simulink model "model_FS_PSH_IEEE39"  (R2020b)
settings: Solver=ode3  StartTime=0.0  StopTime=300  FixedStep=Ts  RelTol=1e-3
PostLoadFcn:
  | IEEE39BusLineLength;
  | vNomHV = 345E3;fNom=60;load('Dynamicload.mat');
InitFcn:
  | IEEE39BusLineLength;
  | vNomHV = 345E3;fNom=60;load('Dynamicload.mat');
values from neighbouring files (symbols this model uses):
  Rp = 0.05    [IEEE39BusLineLength.m]
  t_sw_off = 220    [MAIN_FS_PSH_IEEE39.m]    (also in MAIN_T_PSH_IEEE39.m; MAIN_VS_PSH.m = 45)
  t_sw_on = 130    [MAIN_FS_PSH_IEEE39.m]    (also in MAIN_T_PSH_IEEE39.m; MAIN_VS_PSH.m = 35)
  TL_10_11_len = 14    [IEEE39BusLineLength.m]
  TL_10_13_len = 14    [IEEE39BusLineLength.m]
  TL_13_14_len = 32    [IEEE39BusLineLength.m]
  TL_14_15_len = 70    [IEEE39BusLineLength.m]
  TL_15_16_len = 31.5    [IEEE39BusLineLength.m]
  TL_16_17_len = 26    [IEEE39BusLineLength.m]
  TL_16_19_len = 61    [IEEE39BusLineLength.m]
  TL_16_21_len = 46    [IEEE39BusLineLength.m]
  TL_16_24_len = 15    [IEEE39BusLineLength.m]
  TL_17_18_len = 26    [IEEE39BusLineLength.m]
  TL_17_27_len = 59    [IEEE39BusLineLength.m]
  TL_1_2_len = 134    [IEEE39BusLineLength.m]
  TL_1_39_len = 105    [IEEE39BusLineLength.m]
  TL_21_22_len = 47    [IEEE39BusLineLength.m]
  TL_22_23_len = 33    [IEEE39BusLineLength.m]
  TL_24_23_len = 88    [IEEE39BusLineLength.m]
  TL_25_26_len = 101    [IEEE39BusLineLength.m]
  TL_26_27_len = 46.5    [IEEE39BusLineLength.m]
  TL_26_28_len = 151    [IEEE39BusLineLength.m]
  TL_26_29_len = 200    [IEEE39BusLineLength.m]
  TL_28_29_len = 48    [IEEE39BusLineLength.m]
  TL_2_25_len = 28    [IEEE39BusLineLength.m]
  TL_2_2_len = 49    [IEEE39BusLineLength.m]
  TL_3_18_len = 42    [IEEE39BusLineLength.m]
  TL_3_4_len = 53    [IEEE39BusLineLength.m]
  TL_4_14_len = 33    [IEEE39BusLineLength.m]
  TL_4_5_len = 32.5    [IEEE39BusLineLength.m]
  TL_5_6_len = 14    [IEEE39BusLineLength.m]
  TL_5_8_len = 32    [IEEE39BusLineLength.m]
  TL_6_11_len = 26.5    [IEEE39BusLineLength.m]
  TL_6_7_len = 25.5    [IEEE39BusLineLength.m]
  TL_7_8_len = 15    [IEEE39BusLineLength.m]
  TL_8_9_len = 93    [IEEE39BusLineLength.m]
  TL_9_39_len = 136    [IEEE39BusLineLength.m]
  Ts = 25e-6    (= 2.5e-05)    [MAIN_FS_PSH_IEEE39.m]    (also in MAIN_T_PSH_IEEE39.m; MAIN_VS_PSH.m = 1e-07)
undefined symbols (not defined in the file or in its folder): D1, Delta, FS_PSH, load15, load16, load18, load20, load21, load23, load24, load25, load26, load27, load28, load29, load3, load39, load4, load7, load8
libraries: powerlib x216, sps_avr x10, powerlib_meascontrol x5, pid_lib x1
(part 3 of 8)

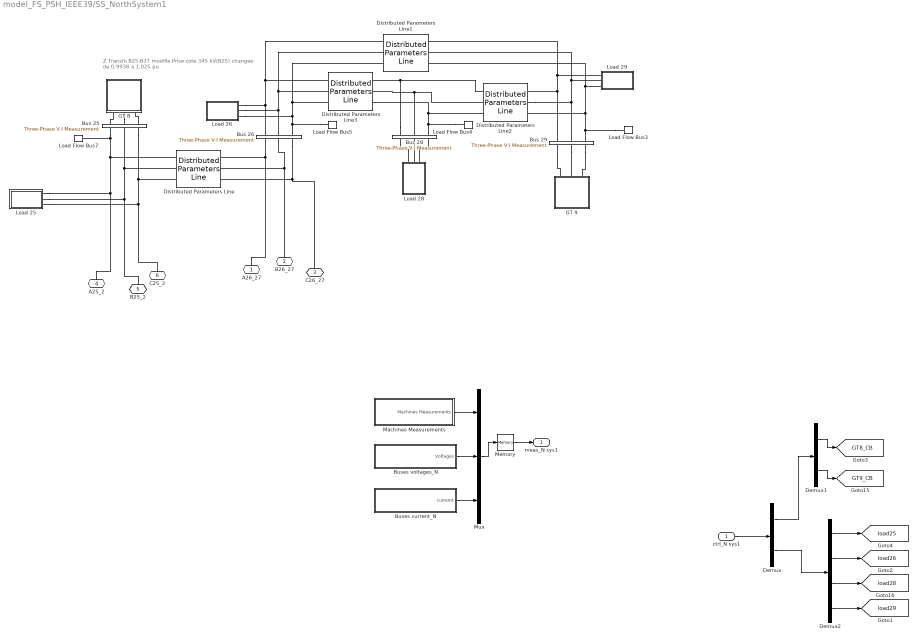
== system model_FS_PSH_IEEE39/SS_NorthSystem1 ==
  note: Z Transfo B25-B37 modifie
      | Prise cote 345 kV(B25)  changee de 0.9938 a 1.025 pu
  ctrl_N sys1 : Inport
  Bus 25 : powerlib/Measurements/Three-Phase V-I Measurement  VoltageMeasurement=phase-to-ground  SetLabelV=on  LabelV=V_bus_25  Vpu=off  VpuLL=off  CurrentMeasurement=yes  SetLabelI=on  LabelI=I_bus_25  Ipu=off  Pbase=100e6  Vbase=230e3  OutputType=Complex  PhasorSimulation=off  PSBequivalent=0
  Bus 26 : powerlib/Measurements/Three-Phase V-I Measurement  VoltageMeasurement=phase-to-ground  SetLabelV=on  LabelV=V_bus_26  Vpu=off  VpuLL=off  CurrentMeasurement=yes  SetLabelI=on  LabelI=I_bus_26  Ipu=off  Pbase=100e6  Vbase=230e3  OutputType=Complex  PhasorSimulation=off  PSBequivalent=0
  Bus 28 : powerlib/Measurements/Three-Phase V-I Measurement  VoltageMeasurement=phase-to-ground  SetLabelV=on  LabelV=V_bus_28  Vpu=off  VpuLL=off  CurrentMeasurement=yes  SetLabelI=on  LabelI=I_bus_28  Ipu=off  Pbase=100e6  Vbase=230e3  OutputType=Complex  PhasorSimulation=off  PSBequivalent=0
  Bus 29 : powerlib/Measurements/Three-Phase V-I Measurement  VoltageMeasurement=phase-to-ground  SetLabelV=on  LabelV=V_bus_29  Vpu=off  VpuLL=off  CurrentMeasurement=yes  SetLabelI=on  LabelI=I_bus_29  Ipu=off  Pbase=100e6  Vbase=230e3  OutputType=Complex  PhasorSimulation=off  PSBequivalent=0
  Buses current_N : Subsystem
  Buses voltages_N : Subsystem
  Demux : Demux  Outputs=[2 8]
  Demux1 : Demux  Outputs=2
  Demux2 : Demux  Outputs=[2 2 2 2]
  Distributed Parameters Line : powerlib/Elements/Distributed Parameters Line  Phases=3  Length=TL_25_26_len  Frequency=fNom  Resistance=[3.809 15.235]/TL_25_26_len  Inductance=[0.102 0.306]/TL_25_26_len  Capacitance=[1.143e-6 0.52e-6]/TL_25_26_len  x1=[-0.0004 -6.49801584942767e-10 0 0;-0.000375 -8.85176084526775e-10 0 0;-0.00035 -1.12047195765278e-09 197383.270025003 -196757.128056257;-0.000325 -1.35566830398082e-09 199228.856843478 -194888.123638832;-0.0003 -1.59074423201149e-09 201056.747002927 -193001.808131403;-0.000275 -1.82567886094164e-09 202866.778139577 -191098.349087419;-0.00025 -2.06045132251909e-09 204658.789475997 -189177.91558312;-0.000225 -2.29504076289635e-09 206432.621835377 -187240.678202513;-0.0002 -2.52942634448289e-09 208188.117655672 -185286.809022224;-0.000175 -2.76358724779611e-09 209925.121003593 -183316.481596211;-0.00015 -2.99750267331064e-09 211643.477588457 -181329.870940347;-0.000125 -3.23115184330587e-09 213343.034775899 -179327.15351688;-0.0001 -3.46451400371154e-09 215023.64160142 -177308.507218749;-7.5e-05 -3.69756842595122e-09 216685.148783807 -175274.111353792;-5e-05 -3.9302944087836e-09 218327.408738383 -173224.146628811;-2.5e-05 -4.16267128014124e-09 219950.275590124 -171158.795133528]  x2=[-0.0004 1.03117190872813e-08 0 0;-0.000375 1.00094674364182e-08 0 0;-0.00035 9.70632668678163e-09 176190.92375866 -212314.939973436;-0.000325 9.40232376508578e-09 178184.078450182 -210644.974463217;-0.0003 9.09748567462794e-09 180161.405801578 -208956.298248395;-0.000275 8.79183949288991e-09 182122.7301752 -207249.061326957;-0.00025 8.48541236913282e-09 184067.877354875 -205523.415345556;-0.000225 8.17823152198559e-09 185996.674561385 -203779.513586048;-0.0002 7.87032423702723e-09 187908.950467809 -202017.510951869;-0.000175 7.56171786436313e-09 189804.535214744 -200237.563954282;-0.00015 7.2524398161957e-09 191683.260425392 -198439.830698471;-0.000125 6.94251756438947e-09 193544.959220518 -196624.470869499;-0.0001 6.63197863803083e-09 195389.466233269 -194791.645718121;-7.5e-05 6.3208506209828e-09 197216.617623868 -192941.518046466;-5e-05 6.00916114943481e-09 199026.251094163 -191074.25219357;-2.5e-05 5.69693790944797e-09 200818.205902046 -189190.014020785]  x3=[-0.0004 7.28520624206915e-11 0 0;-0.000375 7.33520617392959e-11 0 0;-0.00035 7.38455455036475e-11 159.359042835864 -190.278599490576;-0.000325 7.43324698796652e-11 161.14522515065 -188.768251634971;-0.0003 7.48127916159104e-11 162.917093614779 -187.241136291779;-0.000275 7.52864680474291e-11 164.674490840651 -185.697389108214;-0.00025 7.5753457099542e-11 166.417260726082 -184.137147208828;-0.000225 7.62137172915813e-11 168.145248468174 -182.560549183328;-0.0002 7.66672077405753e-11 169.858300577064 -180.967735074265;-0.000175 7.71138881648803e-11 171.55626488956 -179.3588463646;-0.00015 7.75537188877582e-11 173.238990582652 -177.734025965129;-0.000125 7.79866608409012e-11 174.906328186915 -176.093418201797;-0.0001 7.84126755679015e-11 176.558129599783 -174.43716880287;-7.5e-05 7.8831725227668e-11 178.194248098704 -172.765424885996;-5e-05 7.92437725977868e-11 179.81453835417 -171.078334945138;-2.5e-05 7.9648781077828e-11 181.418856442635 -169.376048837377]  x4=[-0.0004 -5.6133067329239e-11 0 0;-0.000375 -5.73097615568789e-11 0 0;-0.00035 -5.84813652001265e-11 991.580164096685 -1246.13955007551;-0.000325 -5.9647774190372e-11 1003.28050960891 -1236.73892106488;-0.0003 -6.08088849204244e-11 1014.8917379452 -1227.22843775233;-0.000275 -6.19645942537151e-11 1026.41281772913 -1217.60894491398;-0.00025 -6.31147995334587e-11 1037.84272559176 -1207.88129700881;-0.000225 -6.42593985917716e-11 1049.18044626259 -1198.04635810275;-0.0002 -6.53982897587474e-11 1060.42497265972 -1188.10500179193;-0.000175 -6.65313718714872e-11 1071.57530597929 -1178.05811112512;-0.00015 -6.76585442830864e-11 1082.63045578423 -1167.90657852522;-0.000125 -6.87797068715739e-11 1093.58944009221 -1157.65130571007;-0.0001 -6.98947600488058e-11 1104.45128546288 -1147.29320361229;-7.5e-05 -7.10036047693117e-11 1115.21502708433 -1136.83319229839;-5e-05 -7.2106142539092e-11 1125.87970885878 -1126.27220088708;-2.5e-05 -7.3202275424367e-11 1136.44438348754 -1115.61116746666]  x5=0.000398898483326272  V1=ones(3,3)  V2=ones(3,3)  I1=ones(3,3)  I2=ones(3,3)  nHarmo=1  Measurements=None  Decoupling=off  VsMag0=0  VrMag0=0  VsAngle0=0  VrAngle0=0  IsMag0=0  IrMag0=0  IsAngle0=0  IrAngle0=0
  Distributed Parameters Line1 : powerlib/Elements/Distributed Parameters Line  Phases=3  Length=TL_26_29_len  Frequency=fNom  Resistance=[6.784 27.138]/TL_26_29_len  Inductance=[0.197 0.592]/TL_26_29_len  Capacitance=[2.293e-6 1.043e-6]/TL_26_29_len  x1=[-0.0008 1.50051894992801e-08 0 0;-0.000775 1.47207537868238e-08 0 0;-0.00075 1.44350104918993e-08 0 0;-0.000725 1.41479849958782e-08 0 0;-0.0007 1.38597027940247e-08 0 0;-0.000675 1.35701894932309e-08 148922.028977619 -232256.649579684;-0.00065 1.3279470809742e-08 151104.338220983 -230842.799306395;-0.000625 1.29875725668726e-08 153273.225503325 -229408.444240916;-0.0006 1.26945206927124e-08 155428.498171536 -227953.711790957;-0.000575 1.24003412178233e-08 157569.964781837 -226478.731174265;-0.00055 1.21050602729271e-08 159697.435116781 -224983.633407148;-0.000525 1.18087040865849e-08 161810.720202151 -223468.551292834;-0.0005 1.15112989828666e-08 163909.632323747 -221933.619409676;-0.000475 1.12128713790131e-08 165993.985044058 -220378.974099199;-0.00045 1.09134477830898e-08 168063.593218823 -218804.75345399;-0.000425 1.06130547916317e-08 170118.273013478 -217211.097305428;-0.0004 1.03117190872813e-08 172157.841919484 -215598.147211267;-0.000375 1.00094674364182e-08 174182.118770535 -213966.046443061;-0.00035 9.70632668678163e-09 176190.92375866 -212314.939973436;-0.000325 9.40232376508578e-09 178184.078450182 -210644.974463217;-0.0003 9.09748567462794e-09 180161.405801578 -208956.298248395;-0.000275 8.79183949288991e-09 182122.7301752 -207249.061326957;-0.00025 8.48541236913282e-09 184067.877354875 -205523.415345556;-0.000225 8.17823152198559e-09 185996.674561385 -203779.513586048;-0.0002 7.87032423702723e-09 187908.950467809 -202017.510951869;-0.000175 7.56171786436313e-09 189804.535214744 -200237.563954282;-0.00015 7.2524398161957e-09 191683.260425392 -198439.830698471;-0.000125 6.94251756438947e-09 193544.959220518 -196624.470869499;-0.0001 6.63197863803083e-09 195389.466233269 -194791.645718121;-7.5e-05 6.3208506209828e-09 197216.617623868 -192941.518046466;-5e-05 6.00916114943481e-09 199026.251094163 -191074.25219357;-2.5e-05 5.69693790944797e-09 200818.205902046 -189190.014020785]  x2=[-0.0008 7.55362211098819e-09 0 0;-0.000775 7.10605204161126e-09 0 0;-0.00075 6.65785077160409e-09 0 0;-0.000725 6.20905811279503e-09 0 0;-0.0007 5.75971392954299e-09 0 0;-0.000675 5.30985813519648e-09 172202.954349061 -215442.997241187;-0.00065 4.85953068854828e-09 174225.766489807 -213810.479094855;-0.000625 4.40877159028602e-09 176233.102890582 -212158.969065496;-0.0006 3.95762087943915e-09 178224.785248162 -210488.613849781;-0.000575 3.50611862982241e-09 180200.636649801 -208799.561818317;-0.00055 3.05430494647624e-09 182160.481588956 -207091.963002472;-0.000525 2.60221996210443e-09 184104.145980865 -205365.969081047;-0.0005 2.14990383350928e-09 186031.45717802 -203621.733366801;-0.000475 1.69739673802468e-09 187942.243985496 -201859.410792836;-0.00045 1.2447388699473e-09 189836.33667616 -200079.157898834;-0.000425 7.91970436966276e-10 191713.567005747 -198281.132817149;-0.0004 3.39131656591792e-10 193573.768227806 -196465.495258766;-0.000375 -1.13737247417326e-10 195416.775108509 -194632.40649911;-0.00035 -5.66596048626487e-10 197242.423941326 -192782.029363726;-0.000325 -1.01940452149849e-09 199050.552561574 -190914.528213808;-0.0003 -1.4721224449666e-09 200841.000360813 -189030.068931607;-0.000275 -1.92470960600719e-09 202613.608301116 -187128.818905693;-0.00025 -2.3771258032117e-09 204368.218929199 -185210.947016086;-0.000225 -2.8293308503576e-09 206104.676390398 -183276.623619257;-0.0002 -3.28128457997789e-09 207822.826442523 -181326.020532994;-0.000175 -3.73294684692907e-09 209522.516469551 -179359.311021142;-0.00015 -4.18427753195704e-09 211203.595495185 -177376.669778212;-0.000125 -4.6352365452607e-09 212865.914196267 -175378.272913863;-0.0001 -5.08578383005301e-09 214509.324916039 -173364.297937258;-7.5e-05 -5.53587936611902e-09 216133.681677256 -171334.923741301;-5e-05 -5.98548317337072e-09 217738.840195161 -169290.330586741;-2.5e-05 -6.4345553153983e-09 219324.657890292 -167230.700086165]  x3=[-0.0008 9.67658806424509e-11 0 0;-0.000775 9.60264170672028e-11 0 0;-0.00075 9.52784238703564e-11 0 0;-0.000725 9.45219674929924e-11 0 0;-0.0007 9.37571151279402e-11 0 0;-0.000675 9.29839347138093e-11 651.879190253851 -1133.09716308397;-0.00065 9.22024949289546e-11 662.529226151143 -1126.90312906639;-0.000625 9.14128651853763e-11 673.120412371758 -1120.60899699703;-0.0006 9.06151156225538e-11 683.651808145296 -1114.21532595707;-0.000575 8.98093171012161e-11 694.122478012292 -1107.72268386936;-0.00055 8.89955411970469e-11 704.531491907304 -1101.1316474479;-0.000525 8.81738601943275e-11 714.877925241533 -1094.44280214666;-0.0005 8.73443470795155e-11 725.160858984947 -1087.65674210756;-0.000475 8.6507075534762e-11 735.379379747913 -1080.77407010768;-0.00045 8.56621199313671e-11 745.532579862332 -1073.79539750575;-0.000425 8.48095553231728e-11 755.619557462263 -1066.72134418783;-0.0004 8.39494574398973e-11 765.639416564033 -1059.55253851222;-0.000375 8.30819026804079e-11 775.591267145819 -1052.2896172537;-0.00035 8.22069681059345e-11 785.474225226711 -1044.93322554693;-0.000325 8.1324731433225e-11 795.287412945228 -1037.48401682917;-0.0003 8.04352710276418e-11 805.029958637294 -1029.94265278218;-0.000275 7.95386658962011e-11 814.700996913671 -1022.30980327355;-0.00025 7.8634995680555e-11 824.299668736819 -1014.5861462971;-0.000225 7.77243406499171e-11 833.825121497207 -1006.77236791269;-0.0002 7.68067816939327e-11 843.276509089042 -998.869162185301;-0.000175 7.58824003154938e-11 852.652991985431 -990.877231123367;-0.00015 7.49512786234991e-11 861.953737312946 -982.797284616414;-0.000125 7.40134993255613e-11 871.17791892561 -974.630040372008;-0.0001 7.306914572066e-11 880.324717478277 -966.376223852008;-7.5e-05 7.21183016917425e-11 889.393320499412 -958.036568208121;-5e-05 7.11610516982736e-11 898.382922463258 -949.611814216781;-2.5e-05 7.01974807687325e-11 907.292724861391 -941.102710213353]  x4=[-0.0008 -5.32627553331173e-11 0 0;-0.000775 -5.34322521881827e-11 0 0;-0.00075 -5.3597002881658e-11 0 0;-0.000725 -5.37569927794341e-11 0 0;-0.0007 -5.39122076702832e-11 0 0;-0.000675 -5.40626337671213e-11 232.453391057633 -505.849442519053;-0.00065 -5.42082577082325e-11 237.210479576283 -503.636188539323;-0.000625 -5.43490665584566e-11 241.946497688563 -501.378198681252;-0.0006 -5.44850478103371e-11 246.66102471396 -499.075673512555;-0.000575 -5.46161893852332e-11 251.353641880922 -496.728817556831;-0.00055 -5.47424796343917e-11 256.023932364061 -494.337839275396;-0.000525 -5.48639073399826e-11 260.671481321171 -491.902951048765;-0.0005 -5.4980461716095e-11 265.295875930081 -489.42436915779;-0.000475 -5.50921324096952e-11 269.896705425324 -486.902313764445;-0.00045 -5.51989095015465e-11 274.473561134621 -484.337008892274;-0.000425 -5.53007835070902e-11 279.026036515185 -481.728682406488;-0.0004 -5.53977453772882e-11 283.553727189828 -479.077565993727;-0.000375 -5.54897864994264e-11 288.056230982887 -476.383895141479;-0.00035 -5.55768986978802e-11 292.533147955939 -473.647909117166;-0.000325 -5.56590742348405e-11 296.984080443334 -470.869850946885;-0.0003 -5.57363058110009e-11 301.408633087513 -468.049967393826;-0.000275 -5.58085865662062e-11 305.806412874125 -465.188508936352;-0.00025 -5.58759100800619e-11 310.177029166943 -462.285729745747;-0.000225 -5.59382703725042e-11 314.520093742555 -459.341887663643;-0.0002 -5.59956619043312e-11 318.835220824855 -456.357244179117;-0.000175 -5.60480795776954e-11 323.122027119303 -453.332064405459;-0.00015 -5.60955187365559e-11 327.380131846979 -450.266617056629;-0.000125 -5.61379751670922e-11 331.609156778399 -447.161174423385;-0.0001 -5.61754450980789e-11 335.808726267117 -444.016012349098;-7.5e-05 -5.62079252012198e-11 339.978467283088 -440.831410205249;-5e-05 -5.62354125914445e-11 344.118009445805 -437.607650866615;-2.5e-05 -5.62579048271641e-11 348.226985057198 -434.345020686138]  x5=0.000785783685246773  V1=ones(3,3)  V2=ones(3,3)  I1=ones(3,3)  I2=ones(3,3)  nHarmo=1  Measurements=None  Decoupling=off  VsMag0=0  VrMag0=0  VsAngle0=0  VrAngle0=0  IsMag0=0  IrMag0=0  IsAngle0=0  IrAngle0=0
  Distributed Parameters Line2 : powerlib/Elements/Distributed Parameters Line  Phases=3  Length=TL_28_29_len  Frequency=fNom  Resistance=[1.666 6.665]/TL_28_29_len  Inductance=[0.048 0.143]/TL_28_29_len  Capacitance=[0.555e-6 0.252e-6]/TL_28_29_len  x1=[-0.0002 -1.22627753912243e-09 0 0;-0.000175 -1.67405795565669e-09 199382.259554779 -190507.622683492;-0.00015 -2.12168967268375e-09 201168.857786666 -188620.054664454;-0.000125 -2.56913292896627e-09 202937.587037427 -186715.732321541;-0.0001 -3.01634798000704e-09 204688.290198301 -184794.824807674;-7.5e-05 -3.46329510157941e-09 206420.811761712 -182857.502748965;-5e-05 -3.90993459325574e-09 208134.997835076 -180903.938229561;-2.5e-05 -4.35622678193386e-09 209830.696154475 -178934.30477636]  x2=[-0.0002 -3.28128457997789e-09 0 0;-0.000175 -3.73294684692907e-09 209522.516469551 -179359.311021142;-0.00015 -4.18427753195704e-09 211203.595495185 -177376.669778212;-0.000125 -4.6352365452607e-09 212865.914196267 -175378.272913863;-0.0001 -5.08578383005301e-09 214509.324916039 -173364.297937258;-7.5e-05 -5.53587936611902e-09 216133.681677256 -171334.923741301;-5e-05 -5.98548317337072e-09 217738.840195161 -169290.330586741;-2.5e-05 -6.4345553153983e-09 219324.657890292 -167230.700086165]  x3=[-0.0002 2.67643326896294e-12 0 0;-0.000175 1.71222017251387e-12 1315.78655166209 -1164.2244305845;-0.00015 7.47854986768843e-13 1326.70046147759 -1151.77191008628;-0.000125 -2.16576627780281e-13 1337.49652608699 -1139.21708254734;-0.0001 -1.18098900474106e-12 1348.1737865214 -1126.56106316006;-7.5e-05 -2.14529647942984e-12 1358.73129436482 -1113.80497610527;-5e-05 -3.10941339648099e-12 1369.16811183835 -1100.94995445236;-2.5e-05 -4.07325411745533e-12 1379.48331188352 -1087.9971400587]  x4=[-0.0002 -5.82099425675479e-12 0 0;-0.000175 -6.07694386964931e-12 30.1483729405909 -130.796513455747;-0.00015 -6.33235369325182e-12 31.3797081394057 -130.506561579167;-0.000125 -6.587201040585e-12 32.608256011103 -130.205017355186;-0.0001 -6.84146327463389e-12 33.8339074289571 -129.891907568706;-7.5e-05 -7.0951178103567e-12 35.0565535235224 -129.567260031946;-5e-05 -7.34814211669091e-12 36.2760856923032 -129.23110358198;-2.5e-05 -7.60051371855463e-12 37.4923956094008 -128.883468078167]  x5=0.000189831504234676  V1=ones(3,3)  V2=ones(3,3)  I1=ones(3,3)  I2=ones(3,3)  nHarmo=1  Measurements=None  Decoupling=off  VsMag0=0  VrMag0=0  VsAngle0=0  VrAngle0=0  IsMag0=0  IrMag0=0  IsAngle0=0  IrAngle0=0
  Distributed Parameters Line3 : powerlib/Elements/Distributed Parameters Line  Phases=3  Length=TL_26_28_len  Frequency=fNom  Resistance=[5.118 20.472]/TL_26_28_len  Inductance=[0.15 0.449]/TL_26_28_len  Capacitance=[1.739e-6 0.791e-6]/TL_26_28_len  x1=[-0.0006 1.26945206927124e-08 0 0;-0.000575 1.24003412178233e-08 0 0;-0.00055 1.21050602729271e-08 0 0;-0.000525 1.18087040865849e-08 161810.720202151 -223468.551292834;-0.0005 1.15112989828666e-08 163909.632323747 -221933.619409676;-0.000475 1.12128713790131e-08 165993.985044058 -220378.9740992;-0.00045 1.09134477830898e-08 168063.593218823 -218804.75345399;-0.000425 1.06130547916317e-08 170118.273013478 -217211.097305428;-0.0004 1.03117190872813e-08 172157.841919484 -215598.147211267;-0.000375 1.00094674364182e-08 174182.118770535 -213966.046443061;-0.00035 9.70632668678163e-09 176190.92375866 -212314.939973436;-0.000325 9.40232376508578e-09 178184.078450182 -210644.974463217;-0.0003 9.09748567462794e-09 180161.405801578 -208956.298248395;-0.000275 8.79183949288991e-09 182122.7301752 -207249.061326957;-0.00025 8.48541236913282e-09 184067.877354875 -205523.415345556;-0.000225 8.17823152198559e-09 185996.674561385 -203779.513586048;-0.0002 7.87032423702723e-09 187908.950467809 -202017.510951869;-0.000175 7.56171786436313e-09 189804.535214744 -200237.563954282;-0.00015 7.2524398161957e-09 191683.260425392 -198439.830698471;-0.000125 6.94251756438947e-09 193544.959220518 -196624.470869499;-0.0001 6.63197863803083e-09 195389.466233269 -194791.645718121;-7.5e-05 6.3208506209828e-09 197216.617623868 -192941.518046466;-5e-05 6.00916114943481e-09 199026.251094163 -191074.25219357;-2.5e-05 5.69693790944797e-09 200818.205902046 -189190.014020785]  x2=[-0.0006 5.92679287461096e-09 0 0;-0.000575 5.48200731026818e-09 0 0;-0.00055 5.03673480233859e-09 0 0;-0.000525 4.59101490250095e-09 172585.310861128 -215083.277740955;-0.0005 4.14488720217396e-09 174604.715817765 -213447.171400399;-0.000475 3.69839132899952e-09 176608.61137396 -211792.105447905;-0.00045 3.25156694332277e-09 178596.819532125 -210118.226896002;-0.000425 2.80445373466923e-09 180569.163688114 -208425.684428262;-0.0004 2.35709141821934e-09 182525.468646915 -206714.628386093;-0.000375 1.90951973128074e-09 184465.56063821 -204985.210755385;-0.00035 1.46177842975857e-09 186389.267331812 -203237.585153014;-0.000325 1.01390728462413e-09 188296.417852967 -201471.906813189;-0.0003 5.65946078382151e-10 190186.84279754 -199688.33257367;-0.000275 1.17934601537134e-10 192060.374247056 -197887.020861833;-0.00025 -3.30087350941101e-10 193916.845783619 -196068.131680602;-0.000225 -7.78079983152228e-10 195756.092504693 -194231.826594228;-0.0002 -1.22600350180031e-09 197577.951037749 -192378.268713949;-0.000175 -1.6738181197285e-09 199382.259554779 -190507.622683492;-0.00015 -2.1214840594531e-09 201168.857786666 -188620.054664454;-0.000125 -2.56896155669691e-09 202937.587037427 -186715.732321541;-0.0001 -3.01621086392126e-09 204688.290198301 -184794.824807674;-7.5e-05 -3.46319225385664e-09 206420.811761712 -182857.502748965;-5e-05 -3.90986602303151e-09 208134.997835076 -180903.938229562;-2.5e-05 -4.35619249529897e-09 209830.696154475 -178934.30477636]  x3=[-0.0006 1.09004175808783e-10 0 0;-0.000575 1.08161974762935e-10 0 0;-0.00055 1.07310166145085e-10 0 0;-0.000525 1.06448825617801e-10 634.586104640281 -979.077420142733;-0.0005 1.05578029690327e-10 643.785327287468 -973.05320520351;-0.000475 1.04697855711793e-10 652.927365199454 -966.942558052308;-0.00045 1.03808381864341e-10 662.011406327571 -960.746021472142;-0.000425 1.02909687156182e-10 671.036643774762 -954.464145875218;-0.0004 1.02001851414575e-10 680.002275867251 -948.09748925405;-0.000375 1.01084955278741e-10 688.907506225756 -941.646617131892;-0.00035 1.00159080192695e-10 697.751543836226 -935.112102512505;-0.000325 9.9224308398017e-11 706.533603120104 -928.49452582926;-0.0003 9.82807229265421e-11 715.252904004103 -921.794474893583;-0.000275 9.73284075929878e-11 723.908671989505 -915.012544842738;-0.00025 9.63674469875085e-11 732.500138220949 -908.149338086965;-0.000225 9.53979264681815e-11 741.026539554726 -901.205464255973;-0.0002 9.44199321534253e-11 749.48711862657 -894.181540144786;-0.000175 9.34335509143496e-11 757.881123918928 -887.078189658955;-0.00015 9.24388703670395e-11 766.207809827715 -879.896043759143;-0.000125 9.14359788647726e-11 774.466436728542 -872.635740405078;-0.0001 9.0424965490171e-11 782.656271042416 -865.297924498882;-7.5e-05 8.94059200472883e-11 790.7765853009 -857.883247827793;-5e-05 8.83789330536329e-11 798.826658210727 -850.392369006264;-2.5e-05 8.73440957321279e-11 806.805774717876 -842.825953417467]  x4=[-0.0006 -7.38334895227681e-11 0 0;-0.000575 -7.39241870212165e-11 0 0;-0.00055 -7.40083181459366e-11 0 0;-0.000525 -7.40858754239154e-11 346.230504208944 -603.710629108254;-0.0005 -7.41568519660671e-11 351.904845857175 -600.420716466848;-0.000475 -7.42212414678448e-11 357.547929282249 -597.077470985713;-0.00045 -7.42790382098007e-11 363.159253232865 -593.681189631243;-0.000425 -7.43302370580939e-11 368.738319278786 -590.232174080785;-0.0004 -7.43748334649467e-11 374.284631855107 -586.730730695844;-0.000375 -7.44128234690484e-11 379.797698306275 -583.177170494867;-0.00035 -7.44442036959072e-11 385.277028929851 -579.571809125618;-0.000325 -7.44689713581499e-11 390.722137020007 -575.914966837139;-0.0003 -7.44871242557694e-11 396.132538910759 -572.206968451308;-0.000275 -7.44986607763205e-11 401.507754018926 -568.448143333981;-0.00025 -7.45035798950628e-11 406.847304886823 -564.638825365739;-0.000225 -7.45018811750515e-11 412.150717224668 -560.77935291223;-0.0002 -7.4493564767177e-11 417.417519952713 -556.870068794112;-0.000175 -7.44786314101506e-11 422.647245243085 -552.911320256605;-0.00015 -7.44570824304393e-11 427.839428561346 -548.903458938645;-0.000125 -7.44289197421483e-11 432.993608707752 -544.846840841646;-0.0001 -7.43941458468503e-11 438.109327858219 -540.741826297885;-7.5e-05 -7.43527638333638e-11 443.186131604994 -536.588779938489;-5e-05 -7.43047773774785e-11 448.223568997014 -532.388070661048;-2.5e-05 -7.42501907416288e-11 453.221192579961 -528.14007159685]  x5=0.00059595217928958  V1=ones(3,3)  V2=ones(3,3)  I1=ones(3,3)  I2=ones(3,3)  nHarmo=1  Measurements=None  Decoupling=off  VsMag0=0  VrMag0=0  VsAngle0=0  VrAngle0=0  IsMag0=0  IrMag0=0  IsAngle0=0  IrAngle0=0
  GT 8 : Subsystem
  GT 9 : Subsystem
  Load 25 : Subsystem  SystemSampleTime=20e-3
  Load 26 : Subsystem  SystemSampleTime=20e-3
  Load 28 : Subsystem  SystemSampleTime=20e-3
  Load 29 : Subsystem  SystemSampleTime=20e-3
  Load Flow Bus3 : powerlib/Measurements/Load Flow Bus  LConnTagsString=a  Phases=single  Connectors=on one side  ID=Bus-29  Vbase=345e+003  Vref=1  Vangle=0  VLF=1.034  VLFb=1  VLFc=1  angleLF=25.68  angleLFb=0  angleLFc=0
      settings: AttributesFormatString=%<ID>\n%<Vbase>V\n%<VLF>pu\n%<angleLF>deg.
  Load Flow Bus4 : powerlib/Measurements/Load Flow Bus  LConnTagsString=a  Phases=single  Connectors=on one side  ID=Bus-28  Vbase=345e+003  Vref=1  Vangle=0  VLF=1.031  VLFb=1  VLFc=1  angleLF=23.66  angleLFb=0  angleLFc=0
      settings: AttributesFormatString=%<ID>\n%<Vbase>V\n%<VLF>pu\n%<angleLF>deg.
  Load Flow Bus5 : powerlib/Measurements/Load Flow Bus  LConnTagsString=a  Phases=single  Connectors=on one side  ID=Bus-26  Vbase=345e+003  Vref=1  Vangle=0  VLF=1.027  VLFb=1  VLFc=1  angleLF=21.79  angleLFb=0  angleLFc=0
      settings: AttributesFormatString=%<ID>\n%<Vbase>V\n%<VLF>pu\n%<angleLF>deg.
  Load Flow Bus7 : powerlib/Measurements/Load Flow Bus  LConnTagsString=a  Phases=single  Connectors=on one side  ID=Bus-25  Vbase=345e+003  Vref=1  Vangle=0  VLF=1.034  VLFb=1  VLFc=1  angleLF=25.05  angleLFb=0  angleLFc=0
      settings: AttributesFormatString=%<ID>\n%<Vbase>V\n%<VLF>pu\n%<angleLF>deg.
  Machines Measurements : Subsystem
      mask Display: disp('Machines Measurements')
  Memory : Memory
  Mux : Mux  Inputs=3
  A26_27 : PMIOPort  Side=Left
  B26_27 : PMIOPort  Port=2  Side=Left
  C26_27 : PMIOPort  Port=3  Side=Left
  A25_2 : PMIOPort  Port=4  Side=Left
  B25_2 : PMIOPort  Port=5  Side=Left
  C25_2 : PMIOPort  Port=6  Side=Left
  meas_N sys1 : Outport
  tag scope: GT8_CB=global, GT9_CB=global, load25=global, load26=global, load28=global, load29=global
  wires:
  Machines Measurements/1(Machines Measurements) -> Mux/1
  Mux/1 -> Memory/1
  Memory/1 -> meas_N sys1/1
  Buses voltages_N/1(Voltages) -> Mux/2
  Buses current_N/1(curremt) -> Mux/3
  ctrl_N sys1/1 -> Demux/1
  Demux/2 -> Demux2/1
  Demux/1 -> Demux1/1
  Demux1/1 -> [GT8_CB]
  Demux1/2 -> [GT9_CB]
  Demux2/1 -> [load25]
  Demux2/2 -> [load26]
  Demux2/3 -> [load28]
  Demux2/4 -> [load29]
  connections:
  Load Flow Bus3/LConn1 -- Load 29/LConn3 -- Distributed Parameters Line1/RConn3 -- Distributed Parameters Line2/RConn3 -- Bus 29/RConn3
  Load 29/LConn2 -- Distributed Parameters Line2/RConn2 -- Bus 29/RConn2 -- Distributed Parameters Line1/RConn2
  Bus 29/LConn3 -- GT 9/RConn3
  Bus 29/LConn2 -- GT 9/RConn2
  GT 9/RConn1 -- Bus 29/LConn1
  Distributed Parameters Line2/LConn2 -- Bus 28/RConn2 -- Distributed Parameters Line3/RConn2
  Load 28/LConn3 -- Bus 28/LConn3
  Load 28/LConn2 -- Bus 28/LConn2
  Load 28/LConn1 -- Bus 28/LConn1
  Bus 25/RConn3 -- GT 8/RConn3
  GT 8/RConn2 -- Bus 25/RConn2
  GT 8/RConn1 -- Bus 25/RConn1
  C25_2/RConn1 -- Bus 25/LConn3 -- Distributed Parameters Line/LConn3 -- Load 25/LConn3
  Load 25/LConn2 -- Bus 25/LConn2 -- Distributed Parameters Line/LConn2 -- B25_2/RConn1
  Load Flow Bus7/LConn1 -- A25_2/RConn1 -- Load 25/LConn1 -- Distributed Parameters Line/LConn1 -- Bus 25/LConn1
  Load Flow Bus5/LConn1 -- Distributed Parameters Line1/LConn3 -- Distributed Parameters Line3/LConn3 -- Load 26/LConn3 -- Bus 26/RConn3
  A26_27/RConn1 -- Bus 26/LConn1 -- Distributed Parameters Line/RConn1
  B26_27/RConn1 -- Bus 26/LConn2 -- Distributed Parameters Line/RConn2
  Bus 26/LConn3 -- C26_27/RConn1 -- Distributed Parameters Line/RConn3
  Load 26/LConn1 -- Distributed Parameters Line1/LConn1 -- Distributed Parameters Line3/LConn1 -- Bus 26/RConn1
  Load 26/LConn2 -- Distributed Parameters Line1/LConn2 -- Distributed Parameters Line3/LConn2 -- Bus 26/RConn2
  Bus 28/RConn1 -- Distributed Parameters Line3/RConn1 -- Distributed Parameters Line2/LConn1
  Load Flow Bus4/LConn1 -- Distributed Parameters Line3/RConn3 -- Distributed Parameters Line2/LConn3 -- Bus 28/RConn3
  Load 29/LConn1 -- Bus 29/RConn1 -- Distributed Parameters Line2/RConn1 -- Distributed Parameters Line1/RConn1
